simulink library "LIB_ENV"  (Simulink 8.8)
settings: Solver=ode45  StartTime=0.0  StopTime=10.0  RelTol=1e-3  EnableMultiTasking=on
settings Model: Creator=alger  LastModifiedBy=Emily

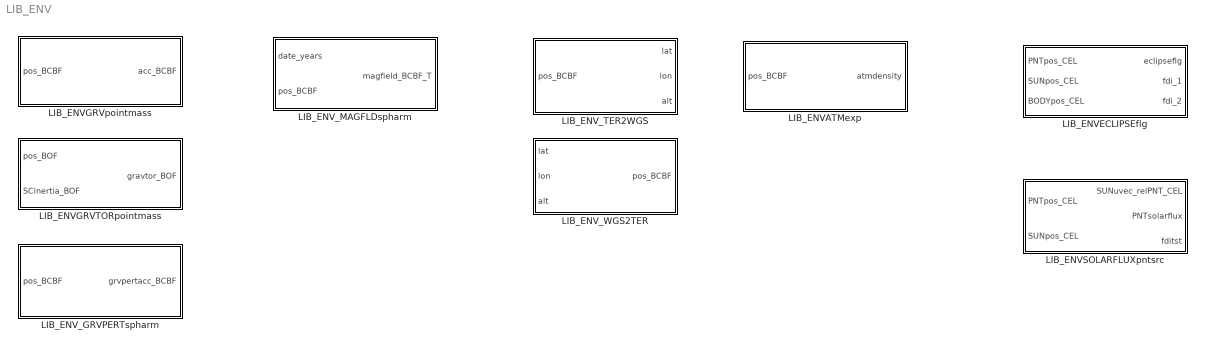
== system LIB_ENV ==
  LIB_ENVATMexp : Subsystem  TreatAsAtomicUnit=on  mask(Computes Density of Atomosphere){rho_ref=9.66e-14, height_ref=71981400, scale_ref=1194800}
      mask prompts: rho_ref "Reference Density (kg/m^3)"; height_ref "Reference distance from earths centre (m)"; scale_ref "Reference Scale height (m)"
      mask help:
      | Computess density of atmosphere at a given location based on exponential model of the atmosphere.
      |
      | Inputs
      |   pos_BCBF: position of the spacecraft in the body centred fixed frame [m]
      |
      | Outputs:
      |    density: density of atmosphere at a given location (kg/m^3)
  LIB_ENVECLIPSEflg : Subsystem  TreatAsAtomicUnit=on  mask(Computes Density of Atomosphere){SUNradius=695700000, BODYradius=6378137, zero_tol=1}
      mask prompts: SUNradius "radius of the Sun (m)"; BODYradius "radius of the celestial body (m)"; zero_tol "tolerance on vector magnitude to prevent division by zero (m)"
      mask help:
      | Calculates the eclipse condition of a point in space w.r.t. the sun body and a generic celestial body.
      |
      | Inputs:
      |   PNTpos_CEL  position to determine eclipse status in a inertial frame (m)
      |   SUNpos_CEL  position of the Sun in a inertial frame (m)
      |   BODYpos_CEL position of the celestial body (Earth, Moon, etc.) in a inertial frame (m)
      |   SUNradius   radius of the Sun (m)
      |   BODYradius  radius of the celestial body (m)
      |   zero_tol    tolerance on vector magnitude to prevent division by zero (m)
      |
      | Outputs:
      |   eclipseflg  eclipse condition
      |                  0: point is in sunlight
      |                  1: point is in umbra
      |                  2: point is in penumbra
      |   fditst      error detection
      |                  0: no problem
      |                  1: either PNTrelBODY_CEL or SUNrelBODY_CEL is a null vector
  LIB_ENVGRVTORpointmass : Subsystem  TreatAsAtomicUnit=on  mask{mu_cst=0}
      mask prompts: mu_cst "body's gravitational parameter [m^3/s^2]"
      mask help:
      | Calculates the gravity gradient torque caused by a point mass for a given orbital position.
      |
      | Inputs:
      |   pos_BOF: position of the spacecraft to the body expressed in the spacecraft body frame [m]
      |   SCinertia_BOF: spacecraft's intertia tensor in BOF frame [kgm^2]
      | Outputs:
      |    grvtor   torque due to gravity gradient expressed in spacecraft body frame [Nm]
  LIB_ENVGRVpointmass : Subsystem  TreatAsAtomicUnit=on  mask(Computes acceleration due to gravity from a point mass){mu_cst=0}
      mask prompts: mu_cst "body's gravitational parameter [m^3/s^2]"
      mask help:
      | Calculates the gravitational acceleration caused by a point mass at a given location.
      |
      | Inputs
      |   pos_BCBF: position of the spacecraft in the body centred fixed frame [m]
      |
      | Outputs:
      |    acc_BCBF: acceleration due to gravity expressed in body centered body fixed frame [m/s^2]
  LIB_ENVSOLARFLUXpntsrc : Subsystem  TreatAsAtomicUnit=on  mask(Compute Solar Flux at a Given Position in Space){solar_flux_ref=1367, solar_dist_ref=149597870700.0, zero_tol=695700000*5}
      mask prompts: solar_flux_ref "reference value to use for the average solar flux (W/m^2)"; solar_dist_ref "distance used to calculate the reference value (m)"; zero_tol "zero tolerence to use on norm (m)"
      mask help:
      | Computes solar flux using a point source approximation for the Sun using the(inverse square law. This approximation is valid for positions  at least 5 Sun diameters away from the Sun.
      |
      | Inputs:
      |   PNTpos_CEL      The point to calculate the solar flux and Sun direction for expressed in CEL frame (m)
      |   SUNpos_CEL      Sun position in CEL frame (m)
      |   solar_flux_ref  The reference value to use for the average solar flux (W/m^2)
      |   solar_dist_ref  The distance used to calculate the reference value (m)
      |
      | Outputs:
      |   PNTsolar_flux       The solar flux from the Sun at this point (W/m^2)
      |   SUNuvec_relPNT_CEL  Unit vector describing the direction between the satellite and the Sun in CEL frame
  LIB_ENV_GRVPERTspharm : Subsystem  TreatAsAtomicUnit=on  mask(Computes non spherical gravity gradient perturbations){mu_cst=0, re_cst=0, maxDegree=0, maxOrder=0, Cnm=0, Snm=0}
      mask prompts: mu_cst "the body's Gravitational constant used to generate Cnm and Snm data [m^3/s^2]"; re_cst "mean radius associated with Cnm and Snm data [m]"; maxDegree "the maximum degree to consider when calculating magnetic field (0-30)[-]"; maxOrder "the maximum order to consider when computeing gravity perturbations (0-30)[-]"; Cnm "non normalized spherical harmonic data  (Zonal components) [30x30][-]"; Snm "non normalized spherical harmonic data (Tesseral/Sectorial components)[30x30][-]"
      mask help:
      | Calculates the gravitational acceleration caused by a point mass at a given location.
      |
      | Inputs
      |   pos_BCBF: position of the spacecraft in the body centred fixed frame [m]
      |
      | Outputs
      |   grvpertacc_BCBF: differences in acceleration due to perturbations from point mass model expressed in body centered body fixed frame [m/s^2]
  LIB_ENV_MAGFLDspharm : Subsystem  TreatAsAtomicUnit=on  mask(Computes magnetic field at a given time or date){maxDegree=0, re_cst=0, Gnm=0, Hnm=0, Gnm_dot=0, Hnm_dot=0, basedate_years=0}
      mask prompts: maxDegree "the maximum degree to consider when calculating magnetic field [-]"; re_cst "radius used to generate zonal, tesseral and sectorial harmonics. [m]"; Gnm "zonal harmonic coefficients at a given basedate[-]"; Hnm "sectorial/tesseral harmonic coefficients at a given basedate[-]"; Gnm_dot "rate of change of zonal harmonic coefficients per year[-]"; Hnm_dot "rate of change of sectorial/tesseral harmonic coefficients per year[-]"; basedate_years "date for which Gnm and Hnm are most valid for in decimal years [years]"
      mask help:
      | Calculates the magnetic field at a given location using either IGRF or WMM data and spherical harmonics modle.
      |
      | Inputs:
      |   date_years: gregorian date in years relative to B.C.E. epoch e.g.(2015.234) [years]
      |   pos_BCBF: position of the spacecraft in the body centred fixed frame [m]
      |
      | Outputs:
      |    magfld_BCBF: magnetic field in tesla expressed in body centered body fixed frame [T]
  LIB_ENV_TER2WGS : Subsystem  TreatAsAtomicUnit=on  mask(Converts position in ECEF to WGS style lat long alt){f=1/298.257223563, r_body=6378137.0, zero_tol=10e-9, maxitterations=5}
      mask prompts: f "flattening constant i.e. 1/298.257223563 [-]"; r_body "equatorial radius of the body [m]"; zero_tol "Near zero tolerence"; maxitterations "maximum number of itterations to limit solution to."
      mask help:
      | Converts postion expressed in  BCBF to WGS coordinates, accounting for
      | earth flatting.
      |
      | Inputs:
      |   pos_BCBF: position in body centred body fixed frame [m]
      |
      | Outputs:
      |   lat: latitude of position [rad]
      |   lon: longitude of postion [rad]
      |   alt: altitude [m]
      |
      | uses ter2wgs() function
  LIB_ENV_WGS2TER : Subsystem  TreatAsAtomicUnit=on  mask(Converts position WGS style lat long alt to position expressed ECEF){f=1/298.257223563, r_body=6378137.0}
      mask prompts: f "flattening constant i.e. 1/298.257223563 [-]"; r_body "equatorial radius of the body [m]"
      mask help:
      | Converts postion expressed in WGS to BCBF coordinates, accounting for  earth flatting.
      |
      | Inputs:
      |   lat: latitude of position [rad]
      |   lon: longitude of postion [rad]
      |   alt: altitude [m]
      |
      | Outputs:
      |   pos_BCBF: position in body centred body fixed frame [m]
      |
      |
      | uses wgs2ter() function

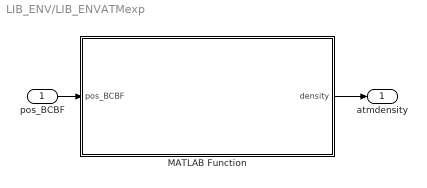
== system LIB_ENV/LIB_ENVATMexp ==
  pos_BCBF : Inport
  MATLAB Function : MATLAB Function  TreatAsAtomicUnit=on
  "atmdensity " : Outport  PortDimensions=1
  wires:
  MATLAB Function/1(density) -> "atmdensity "/1
  pos_BCBF/1 -> MATLAB Function/1(pos_BCBF)

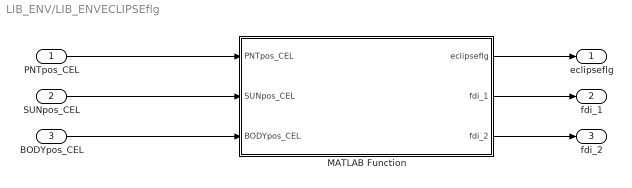
== system LIB_ENV/LIB_ENVECLIPSEflg ==
  PNTpos_CEL : Inport
  SUNpos_CEL : Inport  Port=2
  BODYpos_CEL : Inport  Port=3
  MATLAB Function : MATLAB Function  TreatAsAtomicUnit=on
  "eclipseflg " : Outport  PortDimensions=1
  fdi_1 : Outport  Port=2  PortDimensions=1
  fdi_2 : Outport  Port=3  PortDimensions=1
  wires:
  PNTpos_CEL/1 -> MATLAB Function/1(PNTpos_CEL)
  MATLAB Function/1(eclipseflg) -> "eclipseflg "/1
  MATLAB Function/2(fdi_1) -> fdi_1/1
  BODYpos_CEL/1 -> MATLAB Function/3(BODYpos_CEL)
  SUNpos_CEL/1 -> MATLAB Function/2(SUNpos_CEL)
  MATLAB Function/3(fdi_2) -> fdi_2/1

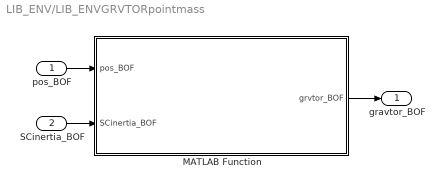
== system LIB_ENV/LIB_ENVGRVTORpointmass ==
  pos_BOF : Inport
  SCinertia_BOF : Inport  Port=2
  MATLAB Function : MATLAB Function  TreatAsAtomicUnit=on
  gravtor_BOF : Outport
  wires:
  MATLAB Function/1(grvtor_BOF) -> gravtor_BOF/1
  pos_BOF/1 -> MATLAB Function/1(pos_BOF)
  SCinertia_BOF/1 -> MATLAB Function/2(SCinertia_BOF)

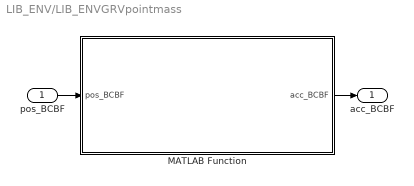
== system LIB_ENV/LIB_ENVGRVpointmass ==
  pos_BCBF : Inport
  MATLAB Function : MATLAB Function  TreatAsAtomicUnit=on
  acc_BCBF : Outport
  wires:
  pos_BCBF/1 -> MATLAB Function/1(pos_BCBF)
  MATLAB Function/1(acc_BCBF) -> acc_BCBF/1

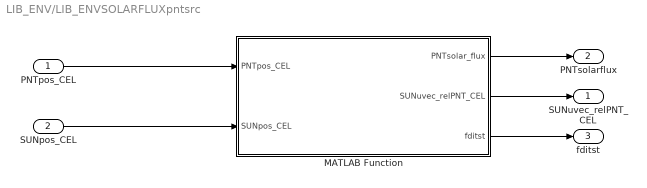
== system LIB_ENV/LIB_ENVSOLARFLUXpntsrc ==
  PNTpos_CEL : Inport  PortDimensions=3
  SUNpos_CEL : Inport  Port=2  PortDimensions=3
  MATLAB Function : MATLAB Function  TreatAsAtomicUnit=on
  SUNuvec_relPNT_CEL : Outport  PortDimensions=3
  "PNTsolarflux " : Outport  Port=2  PortDimensions=1
  fditst : Outport  Port=3  PortDimensions=1
  wires:
  SUNpos_CEL/1 -> MATLAB Function/2(SUNpos_CEL)
  MATLAB Function/2(SUNuvec_relPNT_CEL) -> SUNuvec_relPNT_CEL/1
  MATLAB Function/1(PNTsolar_flux) -> "PNTsolarflux "/1
  PNTpos_CEL/1 -> MATLAB Function/1(PNTpos_CEL)
  MATLAB Function/3(fditst) -> fditst/1

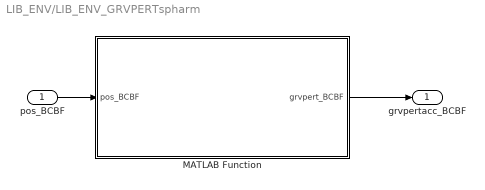
== system LIB_ENV/LIB_ENV_GRVPERTspharm ==
  pos_BCBF : Inport  PortDimensions=3
  MATLAB Function : MATLAB Function  TreatAsAtomicUnit=on
  " grvpertacc_BCBF" : Outport
  wires:
  MATLAB Function/1(grvpert_BCBF) -> " grvpertacc_BCBF"/1
  pos_BCBF/1 -> MATLAB Function/1(pos_BCBF)

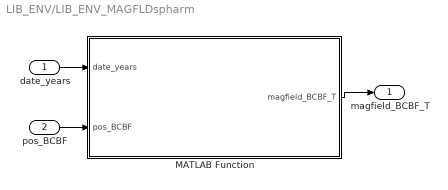
== system LIB_ENV/LIB_ENV_MAGFLDspharm ==
  date_years : Inport  PortDimensions=1
  pos_BCBF : Inport  Port=2  PortDimensions=3
  MATLAB Function : MATLAB Function  TreatAsAtomicUnit=on
  " magfield_BCBF_T" : Outport
  wires:
  pos_BCBF/1 -> MATLAB Function/2(pos_BCBF)
  MATLAB Function/1(magfield_BCBF_T) -> " magfield_BCBF_T"/1
  date_years/1 -> MATLAB Function/1(date_years)

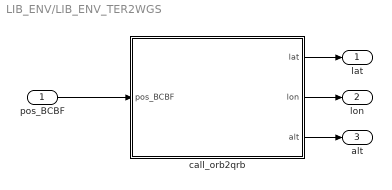
== system LIB_ENV/LIB_ENV_TER2WGS ==
  pos_BCBF : Inport  PortDimensions=3
  call_orb2qrb : MATLAB Function  TreatAsAtomicUnit=on
  lat : Outport  PortDimensions=1
  lon : Outport  Port=2  PortDimensions=1
  alt : Outport  Port=3  PortDimensions=1
  wires:
  call_orb2qrb/1(lat) -> lat/1
  pos_BCBF/1 -> call_orb2qrb/1(pos_BCBF)
  call_orb2qrb/2(lon) -> lon/1
  call_orb2qrb/3(alt) -> alt/1

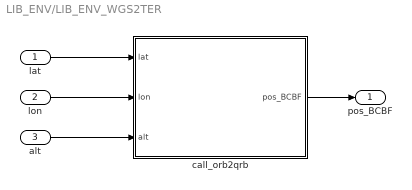
== system LIB_ENV/LIB_ENV_WGS2TER ==
  lat : Inport  PortDimensions=1
  lon : Inport  Port=2  PortDimensions=1
  alt : Inport  Port=3  PortDimensions=1
  call_orb2qrb : MATLAB Function  TreatAsAtomicUnit=on
  "pos_BCBF " : Outport  PortDimensions=3
  wires:
  call_orb2qrb/1(pos_BCBF) -> "pos_BCBF "/1
  lat/1 -> call_orb2qrb/1(lat)
  lon/1 -> call_orb2qrb/2(lon)
  alt/1 -> call_orb2qrb/3(alt)

== matlab function LIB_ENVGRVTORpointmass/MATLAB Function ==
  data: pos_BOF input double; SCinertia_BOF input double; grvtor_BOF output double; mu_cst parameter double
function grvtor_BOF   = call_envgrvtor(pos_BOF, SCinertia_BOF, mu_cst)
%#codegen

[ grvtor_BOF ] = envgrvtor(pos_BOF, SCinertia_BOF, mu_cst);
end

== matlab function LIB_ENVGRVpointmass/MATLAB Function ==
  data: pos_BCBF input double; acc_BCBF output double; mu_cst parameter double
function acc_BCBF   = call_envgrv_pointmass( pos_BCBF, mu_cst )
%#codegen

[ acc_BCBF ] = envgrv_pointmass( pos_BCBF, mu_cst );
end

== matlab function LIB_ENV_MAGFLDspharm/MATLAB Function ==
  data: date_years input double; pos_BCBF input double; magfield_BCBF_T output double; maxDegree parameter double; re_cst parameter double; Gnm parameter double; Hnm parameter double; Gnm_dot parameter double; Hnm_dot parameter double; basedate_years parameter double
function magfield_BCBF_T   = call_envmag_spharm(date_years, pos_BCBF, maxDegree, ...
                                           re_cst, Gnm, Hnm, Gnm_dot, ...
                                           Hnm_dot,  basedate_years)
%#codegen

[magfield_BCBF_T] = envmag_spharm(date_years, pos_BCBF, maxDegree, ...
                                           re_cst, Gnm, Hnm, Gnm_dot, ...
                                           Hnm_dot,  basedate_years);
end

== matlab function LIB_ENV_GRVPERTspharm/MATLAB Function ==
  data: pos_BCBF input double; mu_cst parameter double; re_cst parameter double; grvpert_BCBF output double; maxDegree parameter double; maxOrder parameter double; Cnm parameter double; Snm parameter double
function grvpert_BCBF   = envgrvpert_spharm(pos_BCBF, mu_cst, re_cst, maxDegree, maxOrder, Cnm, Snm)
%#codegen
  [grvpert_BCBF]  =  envgrvpert_spharm(pos_BCBF, mu_cst, re_cst, maxDegree, maxOrder, Cnm, Snm);
end

== matlab function LIB_ENV_TER2WGS/call_orb2qrb ==
  data: pos_BCBF input double; lat output double; f parameter double; r_body parameter double; zero_tol parameter double; maxitterations parameter double; lon output double; alt output double
function [ lat, lon, alt] = call_ter2wgs(pos_BCBF, f, r_body, zero_tol ,maxitterations)
  %#codegen
  [ lat, lon, alt]= ter2wgs(pos_BCBF, f, r_body, zero_tol ,maxitterations);
end

== matlab function LIB_ENV_WGS2TER/call_orb2qrb ==
  data: pos_BCBF output double; lat input double; lon input double; alt input double; f parameter double; r_body parameter double
function pos_BCBF  = call_wgs2ter(lat, lon, alt, f, r_body)
  %#codegen
  [ pos_BCBF]= wgs2ter(lat, lon, alt, f, r_body);
end

== matlab function LIB_ENVATMexp/MATLAB Function ==
  data: pos_BCBF input double; density output double; rho_ref parameter double; height_ref parameter double; scale_ref parameter double
function density  = call_envatm_exp(pos_BCBF, rho_ref, height_ref, scale_ref)
%#codegen

[density] = envatm_exp(pos_BCBF, rho_ref, height_ref, scale_ref);
end

== matlab function LIB_ENVECLIPSEflg/MATLAB Function ==
  data: PNTpos_CEL input double; SUNpos_CEL input double; BODYpos_CEL input double; eclipseflg output double; SUNradius parameter double; BODYradius parameter double; fdi_1 output double; zero_tol parameter double; fdi_2 output double
function [eclipseflg, fdi_1,fdi_2] = call_enveclipse_flg(PNTpos_CEL,     ...
                                                    SUNpos_CEL,     ...
                                                    BODYpos_CEL,    ...
                                                    SUNradius,      ...
                                                    BODYradius,     ...
                                                    zero_tol) 
  %#codegen
  [eclipseflg, fdi_1,fdi_2] = enveclipse_flg(PNTpos_CEL,     ...
                                        SUNpos_CEL,     ...
                                        BODYpos_CEL,    ...
                                        SUNradius,      ...
                                        BODYradius,     ...
                                        zero_tol);
end

== matlab function LIB_ENVSOLARFLUXpntsrc/MATLAB Function ==
  data: PNTpos_CEL input double; SUNpos_CEL input double; PNTsolar_flux output double; solar_dist_ref parameter double; SUNuvec_relPNT_CEL output double; solar_flux_ref parameter double; fditst output double; zero_tol parameter double
function [ PNTsolar_flux, SUNuvec_relPNT_CEL,fditst] = envsolarflux_pntsrc(...
    PNTpos_CEL, ...
    SUNpos_CEL, ...
    solar_dist_ref, solar_flux_ref, zero_tol)
  
  [PNTsolar_flux, SUNuvec_relPNT_CEL,fditst] = envsolarflux_pntsrc(...
    PNTpos_CEL, ...
    SUNpos_CEL, ...
    solar_flux_ref,...
    solar_dist_ref,...
    zero_tol);
end
